simulink model "Practice_verify_battery_current"  (R2014a)
settings: Solver=ode3  StartTime=0.0  StopTime=3600  RelTol=1e-3
undefined symbols (not defined in the file or in its folder): Ion, Lithium
libraries: powerlib x3, electricdrivelib x1
settings Model: Creator=Administrator  LastModifiedBy=Administrator

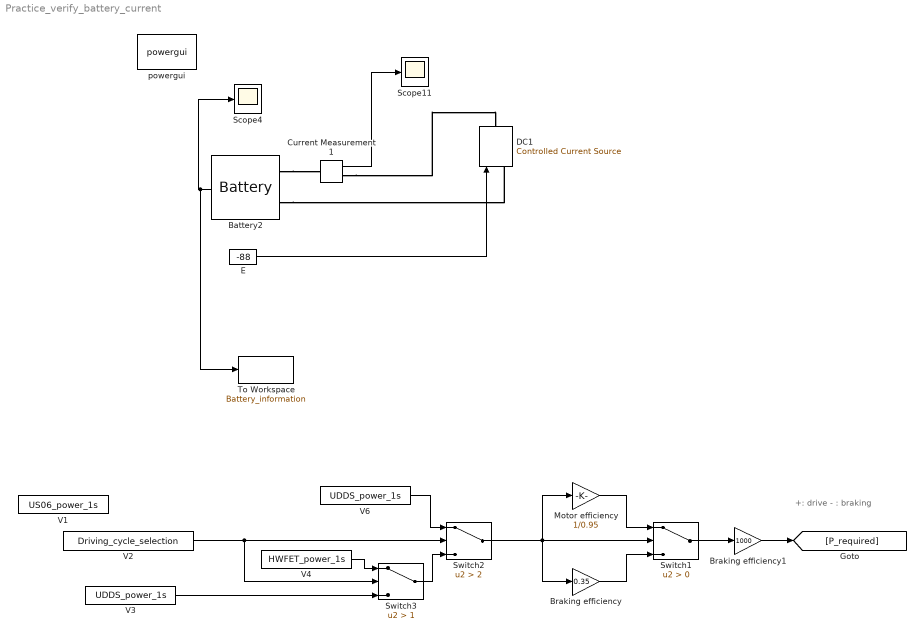
== system Practice_verify_battery_current ==
  note: +: drive
      | - : braking
  Battery2 : electricdrivelib/Extra Sources/Battery  BatType=Lithium-Ion  ShowDetailedParameters=on  NomV=259.25  NomQ=88  SOC=100  PresetModel=on  MaxQ=88  FullV=301.7637  Dis_rate=38.2609  R=0.02946  Normal_OP=79.5826  expZone="[280.09      4.323478]"  Dis_Char=off  current=[1.5 3]  Units=Ampere-hour  Batt_Tr=30
  Braking efficiency : Gain  Gain=0.35
  Braking efficiency1 : Gain  Gain=1000
  Current Measurement1 : powerlib/Measurements/Current Measurement  PhasorSimulation=off  OutputType=Complex  PSBequivalent=0
  DC1 : powerlib/Electrical Sources/Controlled Current Source  Initialize=on  Source_Type=AC  Amplitude=0  Phase=0  Frequency=0  Measurements=None
  E : Constant  Value=-88
  Motor efficiency : Gain  Gain=1/0.95
  Scope11 : Scope
      settings: YMin=409  YMax=419.5  SaveName=ScopeData13
  Scope4 : Scope
      settings: SaveName=ScopeData3
  Switch1 : Switch  Criteria=u2 > Threshold
  Switch2 : Switch  Criteria=u2 > Threshold  Threshold=2
  Switch3 : Switch  Criteria=u2 > Threshold  Threshold=1
  To Workspace : ToWorkspace  VariableName=Battery_information  SampleTime=-1
  V1 : FromWorkspace  VariableName=US06_power_1s  SampleTime=1
  V2 : FromWorkspace  VariableName=Driving_cycle_selection
  V3 : FromWorkspace  VariableName=UDDS_power_1s  SampleTime=1
  V4 : FromWorkspace  VariableName=HWFET_power_1s  SampleTime=1
  V6 : FromWorkspace  VariableName=UDDS_power_1s  SampleTime=1
  powergui : powerlib/powergui  Priority=1  SimulationMode=Discrete  SolverType=Tustin  SampleTime=1  frequency=60  SPID=off  DisableSnubberDevices=off  DisableRonSwitches=off  DisableVfSwitches=off  SwTol=0  Interpol=off  DisplayEquations=off  Ts=0  methode=off  frequencyindice=0  Pbase=100e6  ErrMax=1e-4  Iterations=50  UnitsV=kV  UnitsW=MW  FunctionMessages=off  echomessages=off  HookPort=off  EnableUseOfTLC=off  x0status=blocks  RestoreLinks=warning  ResistiveCurrentMeasurement=off  Frange=[0:2:500]  Ylog=off  Xlog=on  ShowGrid=off  save=off  variable=ZData  structure=0  ZoomFFT=off  StartTime=0.0  cycles=1  DisplayStyle=1  fundamental=60  FreqAxis=off  MaxFrequency=1000  frequencyindicesteady=1  RmsSteady=1  display=off
  wires:
  Battery2/1 -> To Workspace/1, Scope4/1
  E/1 -> DC1/1
  Current Measurement1/1 -> Scope11/1
  Switch2/1 -> Braking efficiency/1, Motor efficiency/1, Switch1/2
  Motor efficiency/1 -> Switch1/1
  Braking efficiency/1 -> Switch1/3
  Switch1/1 -> Braking efficiency1/1
  Braking efficiency1/1 -> [P_required]
  V2/1 -> Switch2/2, Switch3/2
  V3/1 -> Switch3/3
  V4/1 -> Switch3/1
  V6/1 -> Switch2/1
  Switch3/1 -> Switch2/3
  connections:
  Current Measurement1/RConn1 -- DC1/RConn1
  Battery2/LConn2 -- DC1/LConn1
  Battery2/LConn1 -- Current Measurement1/LConn1
